simulink model "Assignment_1_simulation"  (R2022a)
settings: Solver=FixedStepDiscrete  StartTime=0.0  StopTime=360  FixedStep=1  RelTol=1e-3
undefined symbols (not defined in the file): DiscIntNeverNeededParam
settings Model: Creator=anton  LastModifiedBy=anton

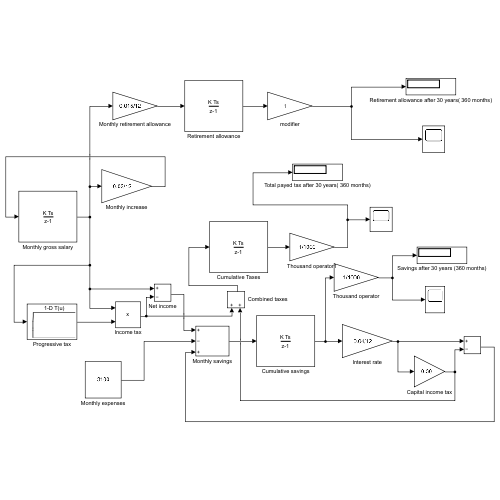
[thumbnail: Simulink's stored preview of the top-level diagram]
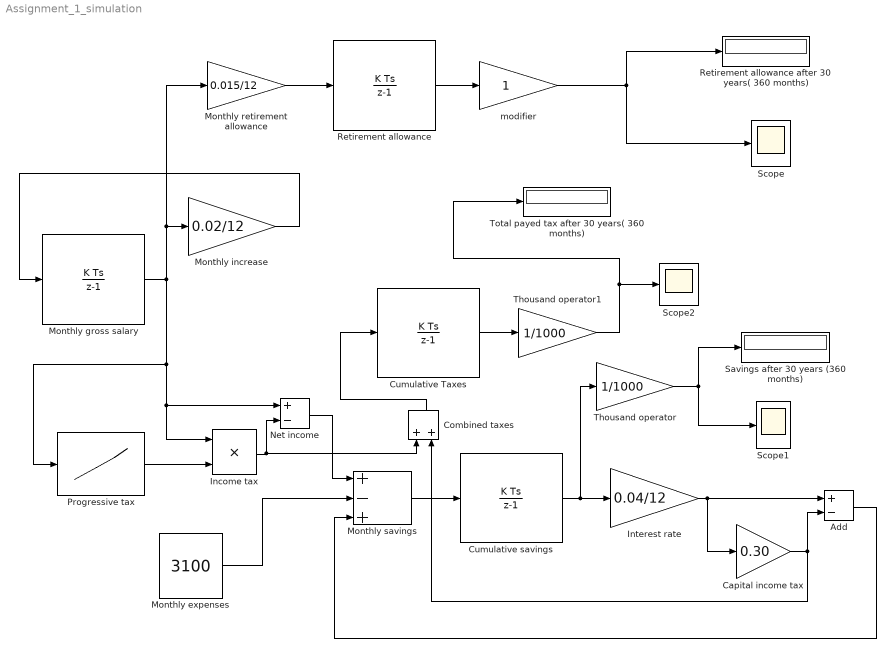
== system Assignment_1_simulation ==
  Add : Sum  Inputs=+-
  Capital income tax : Gain  Gain=0.30
  Combined taxes : Sum
  Cumulative Taxes : DiscreteIntegrator  SampleTime=-1  ICPrevOutput=DiscIntNeverNeededParam  ICPrevScaledInput=DiscIntNeverNeededParam
  Cumulative savings : DiscreteIntegrator  SampleTime=-1  ICPrevOutput=DiscIntNeverNeededParam  ICPrevScaledInput=DiscIntNeverNeededParam
  Income tax : Product
  Interest rate : Gain  Gain=0.04/12
  Monthly expenses : Constant  Value=3100
  Monthly gross salary : DiscreteIntegrator  InitialCondition=3600  SampleTime=-1  ICPrevOutput=DiscIntNeverNeededParam  ICPrevScaledInput=DiscIntNeverNeededParam
  Monthly increase : Gain  Gain=0.02/12
  Monthly retirement allowance : Gain  Gain=0.015/12
  Monthly savings : Sum  Inputs=+-+
  Net income : Sum  Inputs=+-
  Progressive tax : Lookup_n-D  NumberOfTableDimensions=1  BreakpointsForDimension1=[1e3,3e3,5e3,7e3,1e4,1e6]  Table=[0,0.17,0.22,0.37,0.58,0.58]  InternalRulePriority=Speed  RndMeth=Simplest
  Retirement allowance : DiscreteIntegrator  SampleTime=-1  ICPrevOutput=DiscIntNeverNeededParam  ICPrevScaledInput=DiscIntNeverNeededParam
  Retirement allowance after 30 years( 360 months) : Display
  Savings after 30 years (360 months) : Display
  Scope : Scope
  Scope1 : Scope
  Scope2 : Scope
  Thousand operator : Gain  Gain=1/1000
  Thousand operator1 : Gain  Gain=1/1000
  Total payed tax after 30 years( 360 months) : Display
  modifier : Gain
  wires:
  Cumulative savings/1 -> Thousand operator/1, Interest rate/1
  Monthly savings/1 -> Cumulative savings/1
  Thousand operator/1 -> Scope1/1, Savings after 30 years (360 months)/1
  Monthly expenses/1 -> Monthly savings/2
  Add/1 -> Monthly savings/3
  Interest rate/1 -> Capital income tax/1, Add/1
  Capital income tax/1 -> Combined taxes/2, Add/2
  Monthly gross salary/1 -> Monthly retirement allowance/1, Monthly increase/1, Net income/1, Income tax/1, Progressive tax/1
  Monthly increase/1 -> Monthly gross salary/1
  Net income/1 -> Monthly savings/1
  Progressive tax/1 -> Income tax/2
  Income tax/1 -> Combined taxes/1, Net income/2
  Combined taxes/1 -> Cumulative Taxes/1
  Cumulative Taxes/1 -> Thousand operator1/1
  Thousand operator1/1 -> Total payed tax after 30 years( 360 months)/1, Scope2/1
  Monthly retirement allowance/1 -> Retirement allowance/1
  Retirement allowance/1 -> modifier/1
  modifier/1 -> Scope/1, Retirement allowance after 30 years( 360 months)/1
